simulink model "UAV"  (R2025b)
settings: Solver=ode3  StartTime=0.0  StopTime=inf  FixedStep=Sim.Ts_fisica  RelTol=1e-3
PostLoadFcn:
  | Init
InitFcn:
  | Init
model workspace (MAT data in the model file):
  Mass = 1
undefined symbols (not defined in the file): DiscIntNeverNeededParam, Drone, DWORK0, DWORK1, DWORK10, DWORK11, DWORK12, DWORK13, DWORK14, DWORK15, DWORK16, DWORK17, DWORK18, DWORK19, DWORK2, DWORK20, DWORK21, DWORK22, DWORK23, DWORK24, DWORK3, DWORK4, DWORK5, DWORK6, DWORK7, DWORK8, DWORK9, F, Light, MIL, Sim
libraries: simulink x35, slpidlib x11, vrlib x4, aerolibwind2 x2, sim3dlib x2, uavsim3dlib x2
(part 2 of 8)

== system UAV/untitledPanel ==
  Display : CustomWebBlock  Tag=HiddenForWebPanel  PanelInfo="{\"height\":100,\"left\":301,\"panelId\":\"panelId-ef2e9d31-e148-4f09-9232-d82a942bc6a5\",\"top\":152,\"type\":\"panelChild\",\"version\":\"2019b\",\"width\":186,\"zIndex\":1500006}"  LabelPosition=Hide  ShowInitialText=on  Configuration="{\"components\":[{\"name\":\"DisplayComponent\",\"settings\":{\"bold\":false,\"font\":\"DSEG7 Classic\",\"fontColor\":[255,0,0],\"fontSize\":\"30.238036717270703\",\"format\":\"Custom\",\"formatString\":\"%.1f\",\"italic\":false,\"position\":[0,-0.06654504387107983,1,1],\"underline\":false}},{\"name\":\"BackgroundImageComponent\",\"settings\":{\"image\":{\"size\":[260,140],\"src\":\"data:image\\/png;base64,iVBORw0KGgoAAAANSUhEUgAAAQQAAACMCAYAAACanNcLAAAAAXNSR0IArs4c6QAAAARnQU1BAACxjwv8YQUAAAAJcEhZcwAADsMAAA7DAcdvqGQAAAGHaVRYdFhNTDpjb20uYWRvYmUueG1wAAAAAAA8P3hwYWNrZXQgYmVnaW49J++7vycgaWQ9J1c1TTBNcENlaGlIenJlU3pOVGN6a2M5ZCc\\/Pg0KPHg6eG1wbWV0YSB4bWxuczp4PSJhZG9iZTpuczptZXRhLyI+PHJkZjpSREYgeG1sbnM6cmRmPSJodHRwOi8vd3d3LnczLm9yZy8xOTk5LzAyLzIyLXJkZi1zeW50YXgtbnMjIj48cmRmOkRlc2NyaXB0aW9uIHJkZjphYm91dD0idXVpZDpmYWY1YmRkNS1iYTNkLTExZGEtYWQzMS1kMzNkNzUxODJmMWIiIHhtbG5zOnRpZmY9Imh0dHA6Ly9ucy5hZG9iZS5jb20vdGlmZi8xLjAvIj48dGlmZjpPcmllbnRhdGlvbj4xPC90aWZmOk9yaWVudGF0aW9uPjwvcmRmOkRlc2NyaXB0aW9uPjwvcmRmOlJERj48L3g6eG1wbWV0YT4NCjw\\/eHBhY2tldCBlbmQ9J3cnPz4slJgLAAABs0lEQVR4Xu3aMQrCUBRFwR+3KAiuUBDcQiCQfcXuFJ80lpKZ8i7g8Iq37Nt6DIAxxm0egOsSBCCCAEQQgAgCEEEAIghABAGIIABZfvlUvD+e8wT8gc\\/7NU+nXAhABAGIIAARBCCCAEQQgAgCEEEAIghABAGIIAARBCCCAEQQgAgCEEEAIghABAGIIAARBCCCAEQQgAgCEEEAIghABAGIIAARBCCCAEQQgAgCEEEAIghABAGIIAARBCCCAEQQgAgCEEEAIghABAGIIAARBCCCAEQQgAgCEEEAIghABAGIIAARBCCCAEQQgAgCEEEAIghABAGIIAARBCCCAEQQgAgCEEEAIghABAGIIAARBCCCAEQQgAgCEEEAIghABAGIIAARBCCCAEQQgAgCEEEAIghABAGIIAARBCCCAEQQgAgCEEEAIghABAGIIAARBCCCAEQQgAgCEEEAIghABAGIIAARBCCCAEQQgAgCEEEAIghABAGIIAARBCCCAEQQgAgCEEEAIghABAGIIAARBCCCAEQQgAgCkGXf1mMegWtyIQARBCCCAEQQgAgCEEEAIghABAGIIAD5AsLVDdx+I\\/3uAAAAAElFTkSuQmCC\",\"srcOrientation\":\"Right\"},\"position\":[0,0,1,1],\"scaleMode\":\"0\"}},{\"name\":\"ForegroundImageComponent\",\"settings\":{\"angle\":0,\"image\":{\"size\":[0,0],\"src\":\"default\"},\"isForeground\":1,\"position\":[0,0,1,1],\"scaleMode\":\"0\"}}],\"derived\":{\"blockParameters\":{\"fixedAspectRatio\":\"on\",\"format\":\"Custom\",\"formatString\":\"%.1f\"}},\"settings\":{\"BindingType\":\"signal\",\"aspectRatio\":1.032258064516129,\"backgroundColor\":[0,0,0,\"1\"],\"backgroundOffset\":0.14,\"backgroundOpacity\":1,\"fixedAspectRatio\":\"on\",\"showBackgroundColor\":false,\"value\":0,\"version\":\"R2023b\"},\"type\":\"Display\"}"
  Lamp : LampBlock  Tag=HiddenForWebPanel  PanelInfo="{\"height\":97,\"left\":634,\"panelId\":\"panelId-ef2e9d31-e148-4f09-9232-d82a942bc6a5\",\"top\":151,\"type\":\"panelChild\",\"version\":\"2019b\",\"width\":101,\"zIndex\":1500002}"  LabelPosition=Hide  DefaultColor=[192.0, 192.0, 192.0]
  Slider Switch1 : CustomTuningWebBlock  Tag=HiddenForWebPanel  PanelInfo="{\"height\":92,\"left\":27,\"panelId\":\"panelId-ef2e9d31-e148-4f09-9232-d82a942bc6a5\",\"top\":153,\"type\":\"panelChild\",\"version\":\"2019b\",\"width\":224,\"zIndex\":1500004}"  LabelPosition=Hide  ShowInitialText=on  Configuration="{\"components\":[{\"name\":\"CustomSwitchStateComponent\",\"settings\":{\"position\":[0,0,1,1],\"states\":[{\"HitRegion\":{\"position\":[0,0.133,0.36,1]},\"Image\":{\"position\":[0,0.10626201153106984,0.7874759769378603,1],\"size\":[0.7874759769378603,1],\"src\":\"data:image\\/png;base64,iVBORw0KGgoAAAANSUhEUgAAAb8AAADfCAYAAABmkN2cAAAAAXNSR0IArs4c6QAAAARnQU1BAACxjwv8YQUAAAAJcEhZcwAADsMAAA7DAcdvqGQAAAGHaVRYdFhNTDpjb20uYWRvYmUueG1wAAAAAAA8P3hwYWNrZXQgYmVnaW49J++7vycgaWQ9J1c1TTBNcENlaGlIenJlU3pOVGN6a2M5ZCc\\/Pg0KPHg6eG1wbWV0YSB4bWxuczp4PSJhZG9iZTpuczptZXRhLyI+PHJkZjpSREYgeG1sbnM6cmRmPSJodHRwOi8vd3d3LnczLm9yZy8xOTk5LzAyLzIyLXJkZi1zeW50YXgtbnMjIj48cmRmOkRlc2NyaXB0aW9uIHJkZjphYm91dD0idX ...(+23076 chars)\",\"srcOrientation\":\"Right\"},\"Label\":{\"color\":[0,0,0],\"icon\":{\"size\":[0,0],\"src\":[],\"srcOrientation\":\"Right\"},\"iconOffset\":0,\"iconPlacement\":\"left\",\"opacity\":1,\"position\":[0.5,-0.02],\"show\":false,\"text\":{\"content\":\"Off\",\"font\":\"Helvetica\"}},\"Value\":0},{\"HitRegion\":{\"position\":[0,0.5,0.37,1]},\"Image\":{\"position\":[0,0.10564808883194532,0.7887038223361094,1],\"size\":[0.7887038223361094,1],\"src\":\"data:image\\/png;base64,iVBORw0KGgoAAAANSUhEUgAAAb0AAADfCAYAAABiZQ2hAAAAAXNSR0IArs4c6QAAAARnQU1BAACxjwv8YQUAAAAJcEhZcwAADsMAAA7DAcdvqGQAAAGHaVRYdFhNTDpjb20uYWRvYmUueG1wAAAAAAA8P3hwYWNrZXQgYmVnaW49J++7vycgaWQ9J1c1TTBNcENlaGlIenJlU3pOVGN6a2M5ZCc\\/Pg0KPHg6eG1wbWV0YSB4bWxuczp4PSJhZG9iZTpuczptZXRhLyI+PHJkZjpSREYgeG1sbnM6cmRmPSJodHRwOi8vd3d3LnczLm9yZy8xOTk5LzAyLzIyLXJkZi1zeW50YXgtbnMjIj48cmRmOkRlc2NyaXB0aW9uIHJkZjphYm91dD0idX ...(+22578 chars)\",\"srcOrientation\":\"Right\"},\"Label\":{\"color\":[0,0,0],\"icon\":{\"size\":[0,0],\"src\":[],\"srcOrientation\":\"Right\"},\"iconOffset\":0,\"iconPlacement\":\"left\",\"opacity\":1,\"position\":[0.5,0.99],\"show\":false,\"text\":{\"content\":\"On\",\"font\":\"Helvetica\"}},\"Value\":1}]}},{\"name\":\"BackgroundImageComponent\",\"settings\":{\"image\":{\"size\":[140,55],\"src\":\"default\",\"srcOrientation\":\"Right\"},\"position\":[0,0,1,1],\"scaleMode\":\"0\"}},{\"name\":\"ForegroundImageComponent\",\"settings\":{\"image\":{\"size\":[0,0],\"src\":\"default\",\"srcOrientation\":[]},\"isForeground\":1,\"position\":[0,0,1,1],\"scaleMode\":\"0\"}}],\"derived\":{\"blockParameters\":{\"StatesJSON\":[{\"Label\":\"Off\",\"Value\":0},{\"Label\":\"On\",\"Value\":1}],\"fixedAspectRatio\":\"on\"}},\"settings\":{\"BindingType\":\"param\",\"backgroundColor\":[0,0,255,\"1\"],\"backgroundOffset\":0.14,\"fixedAspectRatio\":\"on\",\"foregroundColor\":[234,234,234],\"showBackgroundColor\":false,\"variant\":\"slider\",\"version\":\"R2024b\"},\"type\":\"Switch\"}"
  panelInfo : PanelWebBlock  Tag=HiddenForWebPanel  PanelInfo="{\"compacted\":false,\"height\":457,\"isActiveTab\":true,\"labels\":{\"label1792665653\":{\"deleted\":false,\"left\":628,\"settings\":{\"backgroundColor\":\"rgba(0, 0, 0, 0)\",\"bold\":true,\"font\":\"Arial\",\"fontColor\":\"#ffffff\",\"fontSize\":1.91,\"italicized\":false,\"underlined\":false},\"text\":\"STATUS\",\"top\":277},\"label4773231726\":{\"deleted\":false,\"left\":31,\"settings\":{\"backgroundColor\":\"rgba(0, 0, 0, 0)\",\"bold\":true,\"font\":\"Arial\",\"fontColor\":\"#ffffff\",\"fontSize\":1.96,\"italicized\":false,\"underlined\":false},\"text\":\"MAIN POWER\",\"top\":272},\"label8063236901\":{\"deleted\":false,\"left\":306,\"settings\":{\"backgroundColor\":\"rgba(0, 0, 0, 0)\",\"bold\":true,\"font\":\"Arial\",\"fontColor\":\"#ffffff\",\"fontSize\":2.03,\"italicized\":false,\"underlined\":false},\"text\":\"BATT VOLT\",\"top\":271}},\"left\":71,\"name\":\"Panel\",\"panelId\":\"panelId-ef2e9d31-e148-4f09-9232-d82a942bc6a5\",\"popoutData\":{\"height\":558,\"left\":-1072,\"maximized\":false,\"top\":387,\"width\":830},\"popoutMode\":\"window\",\"tabIndex\":0,\"tabbedSetId\":\"tabbedSet5450734720\",\"top\":206,\"type\":\"panel\",\"version\":\"2019b\",\"visible\":true,\"width\":818,\"zIndex\":1500002}"  PanelSnapshot=<binary blob, 310356 chars, not shown>  PanelBackground=data:image/jpeg;base64,/9j/4AAQSkZJRgABAQAAAQABAAD/2wCEAAUFBQUFBQUGBgUICAcICAsKCQkKCxEMDQwNDBEaEBMQEBMQGhcbFhUWGxcpIBwcICkvJyUnLzkzMzlHREddXX0BBQUFBQUFBQYGBQgIBwgICwoJCQoLEQwNDA0MERoQExAQExAaFxsWFRYbFykgHBwgKS8nJScvOTMzOUdER11dff/CABEIC7gLuAMBIgACEQEDEQH/xAAuAAABBQEBAQAAAAAAAAAAAAAAAwQFBgcCAQgBAQAAAAAAAAAAAAAAAAAAAAD/2gAMAwEAAhADEAAAANKZNWI9i+Ghg4AAAAAAABrGT6sbgJ+ndOtdPMU+iPnLeB00ZNR7877zghwAAAAAAABqW04tswrzxyVbEtoxQ+g2 ...(+870532 chars)
